simulink subsystem "ControllerBA"  (R2023b)
settings: Solver=VariableStepAuto  StartTime=0.0  StopTime=10.0  RelTol=1e-3
settings Model: Creator=chaya  LastModifiedBy=chaya

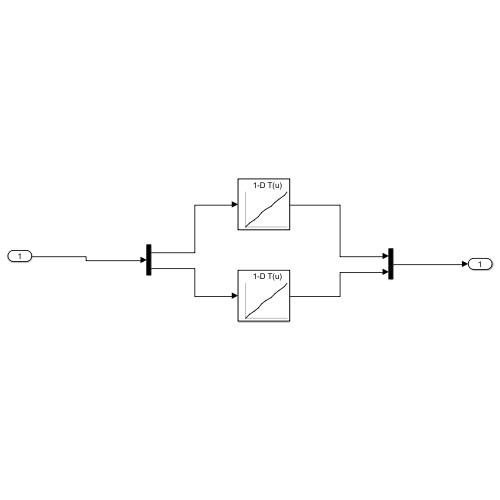
[thumbnail: Simulink's stored preview of the top-level diagram]
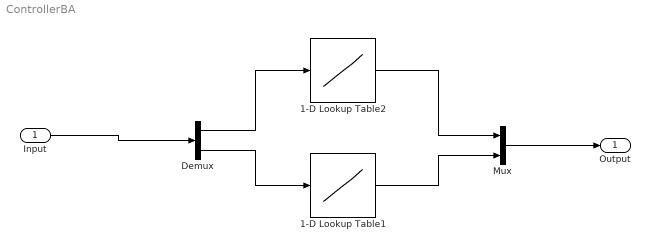
== system ControllerBA ==
  Input : Inport
  1-D Lookup Table1 : Lookup_n-D  NumberOfTableDimensions=1  BreakpointsForDimension1=[-0.434135437011719 -0.350112915039063 -0.252082824707031 -0.168052673339844 -0.0840225219726563 0 0.112030029296875 0.196067810058594 0.280082702636719 0.392127990722656 0.448146820068359]  Table=[-254 -199.389953613281 -149.859985351563 -100.32999420166 -49.5299835205078 0 49.724983215332 99.4500274658203 150.450012207031 200.175018310547 255]  InternalRulePriority=Speed  RndMeth=Simplest
  1-D Lookup Table2 : Lookup_n-D  NumberOfTableDimensions=1  BreakpointsForDimension1=[-0.434135437011719 -0.350112915039063 -0.252082824707031 -0.168052673339844 -0.0840225219726563 0 0.112030029296875 0.196067810058594 0.280082702636719 0.392127990722656 0.448146820068359]  Table=[-254 -199.389953613281 -149.859985351563 -100.32999420166 -49.5299835205078 0 49.724983215332 99.4500274658203 150.450012207031 200.175018310547 255]  InternalRulePriority=Speed  RndMeth=Simplest
  Demux : Demux  Outputs=2
  Mux : Mux  Inputs=2
  Output : Outport
  wires:
  Input/1 -> Demux/1
  Mux/1 -> Output/1
  Demux/1 -> 1-D Lookup Table2/1
  Demux/2 -> 1-D Lookup Table1/1
  1-D Lookup Table1/1 -> Mux/2
  1-D Lookup Table2/1 -> Mux/1
